simulink model "statefdbk"  (R2023a)
settings: Solver=VariableStepAuto  StartTime=0.0  StopTime=3.0  RelTol=1e-3
values from neighbouring files (symbols this model uses):
  A = [A zeros(n,1); -C_ 1]    [control_integral.m]    (also in model.mat = [2.19826062055 1 0 0 0 0 -0.950981109251 0 1 0 0 0 ... (36 e; square_2V_2_5hz_100fs.mat = [3.68944323306 1 0 0 0 0 0 0 0 0 0 -4.87835143564 ... (121 e; square_2V_2_5hz_50fs.mat = [3.32314178319 1 0 0 0 0 0 0 0 0 0 -4.05203564565 ... (121 e)
  B = [B ; 0]    [control_integral.m]    (also in model.mat = [1 0 0 0 0 0]; square_2V_2_5hz_100fs.mat = [1 0 0 0 0 0 0 0 0 0 0]; square_2V_2_5hz_50fs.mat = [1 0 0 0 0 0 0 0 0 0 0])
  C = eye(6)    [control.m]    (also in control_integral.m; model.mat = [-0.0688244704241 0.243744146338 -0.160379964746 0.159733475; square_2V_2_5hz_100fs.mat = [0.0387406639515 -0.00769875135999 -0.0877071898369 0.106733; square_2V_2_5hz_50fs.mat = [0.137657900871 -0.107456657028 -0.0846958769464 0.059459958)
  C_ = C    [control.m]    (also in control_integral.m)
  D = zeros(size(A,1),1)    [control.m]    (also in control_integral.m; model.mat = 0; plotter.m = sign(tensao_gage.signals.values(2))*str2double(strcat(newStr; square_2V_2_5hz_100fs.mat = 0)
  K = dlqr(A,B,Q,R)    [control.m]    (also in control_integral.m = K(1:end-1))
  R_v = 1    [control.m]    (also in control_integral.m)
  x0 = [10 0 0 0 0 10]    [control.m]    (also in control_integral.m = [0 0 0 0 0 0]; model_identification_ecpd.m = findstates(sys,iddata(y,u,1/fs)))
undefined symbols (not defined in the file or in its folder): Discrete, Time
libraries: ctrlSharedLib x1
settings Model: Creator=Tiago  LastModifiedBy=Tiago
settings SolverCC: AlgebraicLoopSolver=TrustRegion
settings DataIOCC: ReturnWorkspaceOutputs=off
settings DebuggingCC: UnconnectedInputMsg=warning  UnconnectedOutputMsg=warning  UnconnectedLineMsg=warning
settings ModelReferenceCC: EnableRefExpFcnMdlSchedulingChecks=on
settings RTWCC: DLArmComputeVersion=19.05

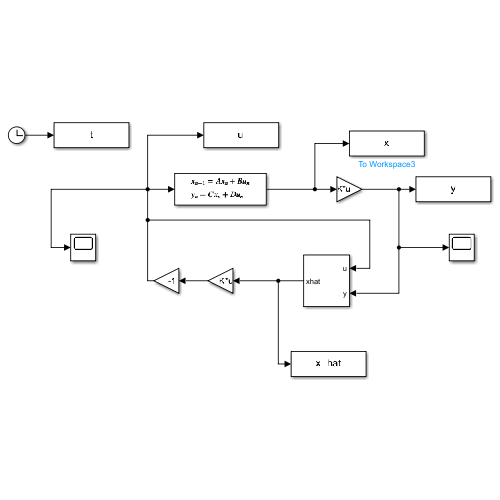
[thumbnail: Simulink's stored preview of the top-level diagram]
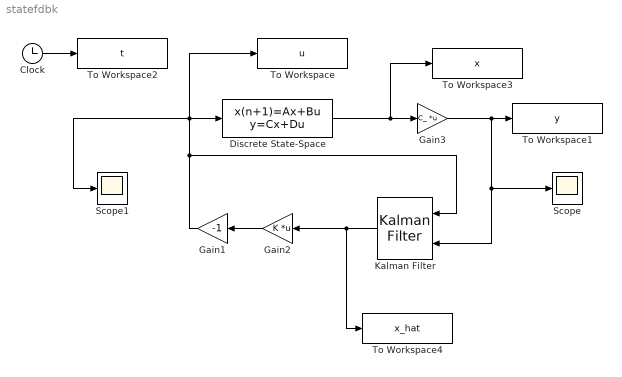
== system statefdbk ==
  Clock : Clock
  Discrete State-Space : DiscreteStateSpace  A=A  B=B  C=C  D=D  InitialCondition=x0  SampleTime=0.02
  Gain1 : Gain  Gain=-1
  Gain2 : Gain  Gain=K  Multiplication=Matrix(K*u)
  Gain3 : Gain  Gain=C_  Multiplication=Matrix(K*u)
  Kalman Filter : ctrlSharedLib/Kalman Filter  TimeDomain=Discrete-Time  UseCurrentEstimator=on  ModelSource=Individual A, B, C, D matrices  ModelSourceVariable=ss(0.95,1,1,0,1)  A=A  B=B  C=C_  D=0  NumberOfStates=1  NumberOfInputs=1  NumberOfOutputs=1  InitialEstimateSource=Dialog  X0=[0 0 0 0 0 0]  P0=10  UseK=off  UseGH=off  NumberOfProcessNoiseInputs=1  G=1  TimeInvariantG=on  H=0  TimeInvariantH=on  Q=Q_w  TimeInvariantQ=on  R=R_v  TimeInvariantR=on  N=0  TimeInvariantN=on  AddInputPort=on  AddEnablePort=off  OutputEstimatedY=off  OutputP=off  Ts=0.02
  Scope : Scope
  Scope1 : Scope
  To Workspace : ToWorkspace  VariableName=u  SaveFormat=Structure  SampleTime=-1
  To Workspace1 : ToWorkspace  VariableName=y  SampleTime=-1
  To Workspace2 : ToWorkspace  VariableName=t  SampleTime=-1
  To Workspace3 : ToWorkspace  VariableName=x  SampleTime=-1
  To Workspace4 : ToWorkspace  VariableName=x_hat  SampleTime=-1
  wires:
  Gain1/1 -> Kalman Filter/1, Scope1/1, Discrete State-Space/1, To Workspace/1
  Clock/1 -> To Workspace2/1
  Gain2/1 -> Gain1/1
  Discrete State-Space/1 -> Gain3/1, To Workspace3/1
  Gain3/1 -> Scope/1, Kalman Filter/2, To Workspace1/1
  Kalman Filter/1 -> To Workspace4/1, Gain2/1
